simulink model "signal_generator"  (R2020b)
settings: Solver=VariableStepAuto  StartTime=0.0  StopTime=2048/(fs*8)  RelTol=1e-3
values from neighbouring files (symbols this model uses):
  aximm_bits = n_blocks * k    (= 800)    [setup.m]
  aximm_enable = 1    [setup.m]
  aximm_reset = 0    [setup.m]
  fs = 160e6    (= 160000000)    [setup.m]
  k = 80    [fixed_point_to_frame.m]    (also in setup.m)
libraries: hdlsllib x12, dspsigops x7, commblkcod2 x1, simulink x1, lib_rfsoc_fec x1
settings Model: SimulationMode=accelerator  Creator=ckb13136  LastModifiedBy=ckb13136
settings GRTTargetCC: RTWCAPISignals=on  RTWCAPIParams=on

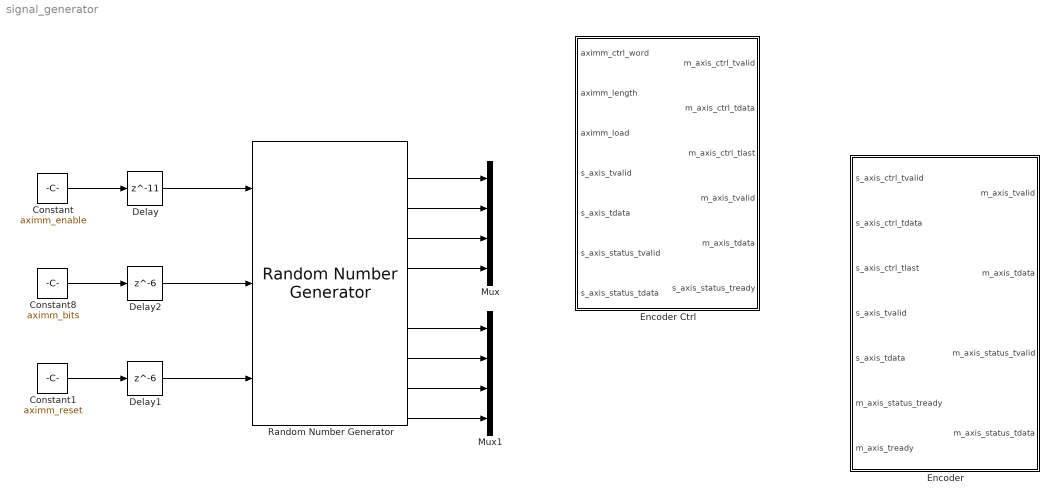
== system signal_generator ==
  Constant : Constant  Value=aximm_enable  OutDataTypeStr=uint32  SampleTime=1/fs
  Constant1 : Constant  Value=aximm_reset  OutDataTypeStr=uint32  SampleTime=1/fs
  Constant8 : Constant  Value=aximm_bits  OutDataTypeStr=uint32  SampleTime=1/fs
  Delay : Delay  DelayLength=11
  Delay1 : Delay  DelayLength=6
  Delay2 : Delay  DelayLength=6
  Encoder : Subsystem
  Encoder Ctrl : Subsystem  AncestorBlock=lib_rfsoc_fec/FEC Ctrl  TreatAsAtomicUnit=on
  Mux : Mux
  Mux1 : Mux
  Random Number Generator : lib_rfsoc_fec/Random Number Generator  SystemSampleTime=-1  VariantActivationTime=update diagram  Latency=0  AutoFrameSizeCalculation=off
  wires:
  Delay/1 -> Random Number Generator/1
  Constant8/1 -> Delay2/1
  Delay2/1 -> Random Number Generator/2
  Constant/1 -> Delay/1
  Delay1/1 -> Random Number Generator/3
  Constant1/1 -> Delay1/1
  Random Number Generator/2 -> Mux/1
  Random Number Generator/3 -> Mux/2
  Random Number Generator/4 -> Mux/3
  Random Number Generator/5 -> Mux/4
  Random Number Generator/7 -> Mux1/1
  Random Number Generator/8 -> Mux1/2
  Random Number Generator/9 -> Mux1/3
  Random Number Generator/10 -> Mux1/4

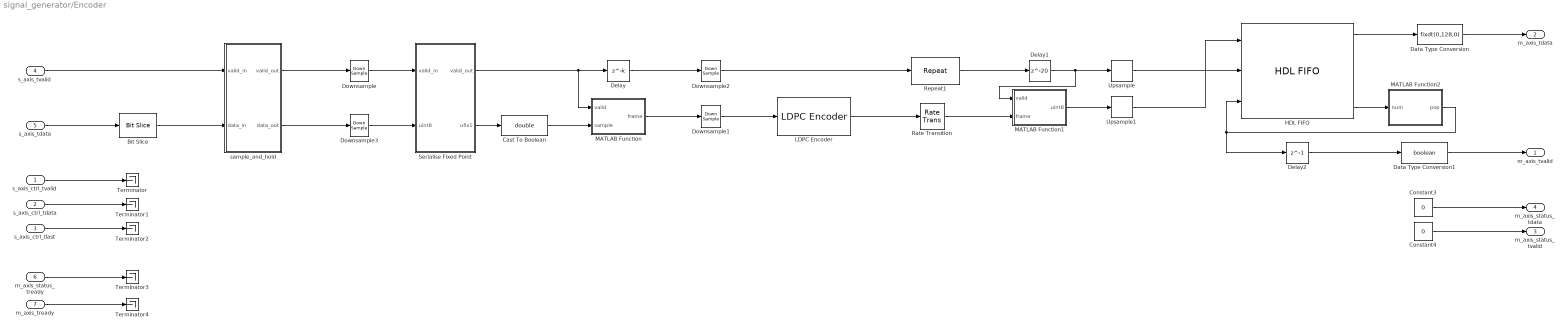
== system signal_generator/Encoder ==
  s_axis_ctrl_tvalid : Inport
  s_axis_ctrl_tdata : Inport  Port=2
  s_axis_ctrl_tlast : Inport  Port=3
  s_axis_tvalid : Inport  Port=4
  s_axis_tdata : Inport  Port=5
  m_axis_status_tready : Inport  Port=6
  m_axis_tready : Inport  Port=7
  Bit Slice : hdlsllib/Logic and Bit Operations/Bit Slice  lidx=7  ridx=0
      settings: SourceProductBaseCode=SL
  Cast To Boolean : DataTypeConversion  OutDataTypeStr=double
  Constant3 : Constant  Value=0  OutDataTypeStr=uint32  SampleTime=1/(fs*16)
  Constant4 : Constant  Value=0  OutDataTypeStr=boolean  SampleTime=1/(fs*16)
  Data Type Conversion : DataTypeConversion  OutDataTypeStr=fixdt(0,128,0)
  Data Type Conversion1 : DataTypeConversion  OutDataTypeStr=boolean
  Delay : Delay  DelayLength=k
  Delay1 : Delay  DelayLength=20
  Delay2 : Delay  DelayLength=1
  Downsample : DownSample  N=16  RateOptions=Allow multirate processing
  Downsample1 : DownSample  N=80  RateOptions=Allow multirate processing
  Downsample2 : DownSample  N=80  RateOptions=Allow multirate processing
  Downsample3 : DownSample  N=16  RateOptions=Allow multirate processing
  HDL FIFO : hdlsllib/HDL RAMs/HDL FIFO  fifo_size=8192  mode=Classic  ratio=1  push_msg=Warning  pop_msg=Warning  show_empty=on  show_full=on  show_num=on  LabelModeActiveChoice_Mode=Classic
      settings: SourceProductBaseCode=SL
  LDPC Encoder : commblkcod2/LDPC Encoder  ParityCheckMat=parity_sparse
      settings: SourceProductBaseCode=CM
  MATLAB Function : MATLAB Function  TreatAsAtomicUnit=on
  MATLAB Function1 : MATLAB Function  TreatAsAtomicUnit=on
  MATLAB Function2 : MATLAB Function  TreatAsAtomicUnit=on
  Rate Transition : RateTransition
  Repeat1 : dspsigops/Repeat  N=20  InputProcessing=Columns as channels (frame based)  RateOptions=Allow multirate processing  ic=0  mode=Unused parameter value
      settings: SourceProductName=DSP System Toolbox
  Serialise Fixed Point : Subsystem
  Terminator{,1..4} (5 alike) : Terminator
  Upsample : dspsigops/Upsample  N=8  phase=0  RateOptions=Allow multirate processing  ic=0  mode=Unused parameter value
  Upsample1 : dspsigops/Upsample  N=8  phase=0  RateOptions=Allow multirate processing  ic=0  mode=Unused parameter value
  sample_and_hold : Subsystem
  m_axis_tvalid : Outport
  m_axis_tdata : Outport  Port=2
  m_axis_status_tvalid : Outport  Port=3
  m_axis_status_tdata : Outport  Port=4
  wires:
  m_axis_tready/1 -> Terminator4/1
  Data Type Conversion1/1 -> m_axis_tvalid/1
  Delay2/1 -> Data Type Conversion1/1
  MATLAB Function2/1(pop) -> HDL FIFO/3, Delay2/1
  HDL FIFO/4 -> MATLAB Function2/1(num)
  Data Type Conversion/1 -> m_axis_tdata/1
  Upsample/1 -> HDL FIFO/2
  Upsample1/1 -> HDL FIFO/1
  HDL FIFO/1 -> Data Type Conversion/1
  Delay1/1 -> Upsample/1, MATLAB Function1/1(valid)
  Bit Slice/1 -> sample_and_hold/2(data_in)
  Rate Transition/1 -> MATLAB Function1/2(frame)
  LDPC Encoder/1 -> Rate Transition/1
  sample_and_hold/2(" data_out") -> Downsample3/1
  sample_and_hold/1(" valid_out") -> Downsample/1
  s_axis_tdata/1 -> Bit Slice/1
  s_axis_tvalid/1 -> sample_and_hold/1(valid_in)
  Downsample3/1 -> Serialise Fixed Point/2(uint8)
  m_axis_status_tready/1 -> Terminator3/1
  s_axis_ctrl_tlast/1 -> Terminator2/1
  s_axis_ctrl_tdata/1 -> Terminator1/1
  s_axis_ctrl_tvalid/1 -> Terminator/1
  Downsample/1 -> Serialise Fixed Point/1(valid_in)
  Downsample1/1 -> LDPC Encoder/1
  Delay/1 -> Downsample2/1
  Repeat1/1 -> Delay1/1
  MATLAB Function1/1(uint8) -> Upsample1/1
  MATLAB Function/1(frame) -> Downsample1/1
  Serialise Fixed Point/1(valid_out) -> MATLAB Function/1(valid), Delay/1
  Cast To Boolean/1 -> MATLAB Function/2(sample)
  Downsample2/1 -> Repeat1/1
  Constant4/1 -> m_axis_status_tvalid/1
  Constant3/1 -> m_axis_status_tdata/1
  Serialise Fixed Point/2(ufix1) -> Cast To Boolean/1

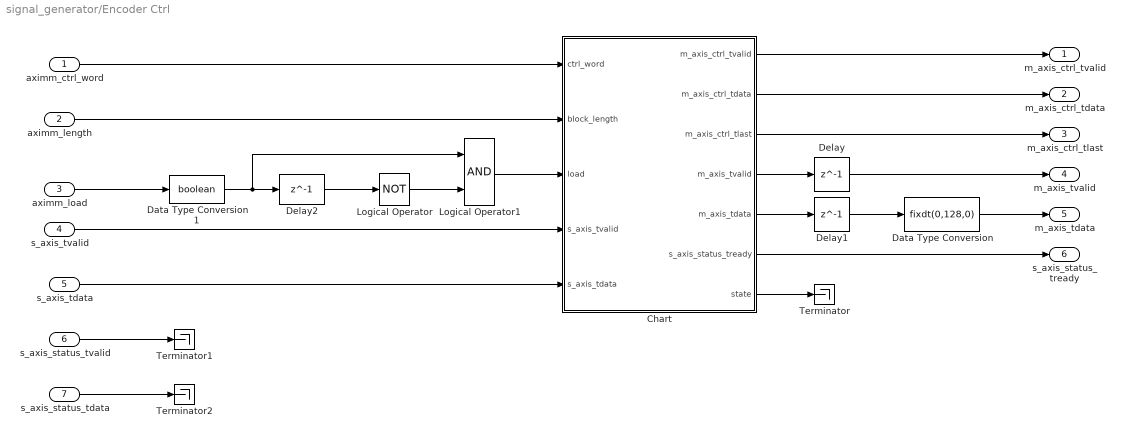
== system signal_generator/Encoder Ctrl ==
  aximm_ctrl_word : Inport
  aximm_length : Inport  Port=2
  aximm_load : Inport  Port=3
  s_axis_tvalid : Inport  Port=4
  s_axis_tdata : Inport  Port=5
  s_axis_status_tvalid : Inport  Port=6
  s_axis_status_tdata : Inport  Port=7
  Chart : Stateflow chart  TreatAsAtomicUnit=on
  Data Type Conversion : DataTypeConversion  OutDataTypeStr=fixdt(0,128,0)
  Data Type Conversion1 : DataTypeConversion  OutDataTypeStr=boolean  SaturateOnIntegerOverflow=on  RndMeth=Zero
  Delay : Delay  DelayLength=1
  Delay1 : Delay  DelayLength=1
  Delay2 : Delay  DelayLength=1  InitialCondition=1  InputProcessing=Columns as channels (frame based)
  Logical Operator : Logic  Operator=NOT  Inputs=1
  Logical Operator1 : Logic
  Terminator : Terminator
  Terminator1 : Terminator
  Terminator2 : Terminator
  m_axis_ctrl_tvalid : Outport
  m_axis_ctrl_tdata : Outport  Port=2
  m_axis_ctrl_tlast : Outport  Port=3
  m_axis_tvalid : Outport  Port=4
  m_axis_tdata : Outport  Port=5
  s_axis_status_tready : Outport  Port=6
  wires:
  Chart/3(m_axis_ctrl_tlast) -> m_axis_ctrl_tlast/1
  Chart/7(state) -> Terminator/1
  aximm_length/1 -> Chart/2(block_length)
  s_axis_tvalid/1 -> Chart/4(s_axis_tvalid)
  s_axis_tdata/1 -> Chart/5(s_axis_tdata)
  aximm_ctrl_word/1 -> Chart/1(ctrl_word)
  Chart/2(m_axis_ctrl_tdata) -> m_axis_ctrl_tdata/1
  Chart/4(m_axis_tvalid) -> Delay/1
  Chart/5(m_axis_tdata) -> Delay1/1
  Chart/6(s_axis_status_tready) -> s_axis_status_tready/1
  Chart/1(m_axis_ctrl_tvalid) -> m_axis_ctrl_tvalid/1
  Delay/1 -> m_axis_tvalid/1
  Delay1/1 -> Data Type Conversion/1
  Data Type Conversion/1 -> m_axis_tdata/1
  Logical Operator1/1 -> Chart/3(load)
  s_axis_status_tvalid/1 -> Terminator1/1
  s_axis_status_tdata/1 -> Terminator2/1
  Logical Operator/1 -> Logical Operator1/2
  Data Type Conversion1/1 -> Delay2/1, Logical Operator1/1
  Delay2/1 -> Logical Operator/1
  aximm_load/1 -> Data Type Conversion1/1

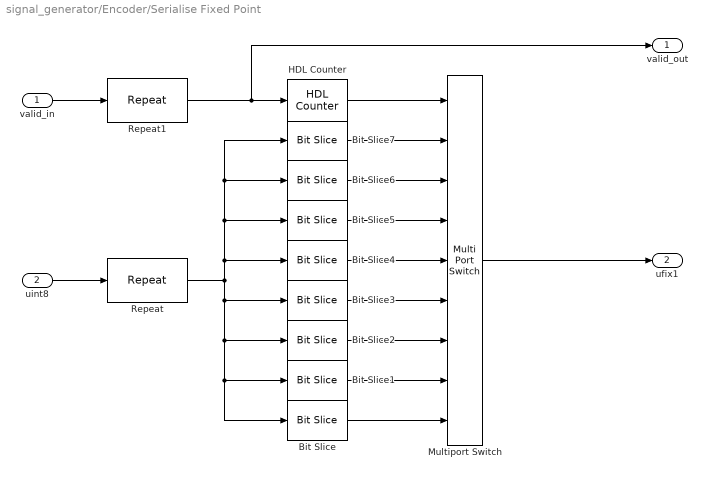
== system signal_generator/Encoder/Serialise Fixed Point ==
  valid_in : Inport
  uint8 : Inport  Port=2
  Bit Slice : hdlsllib/Logic and Bit Operations/Bit Slice  lidx=0  ridx=0
      settings: SourceProductBaseCode=SL
  Bit Slice1 : hdlsllib/Logic and Bit Operations/Bit Slice  lidx=1  ridx=1
      settings: SourceProductBaseCode=SL
  Bit Slice2 : hdlsllib/Logic and Bit Operations/Bit Slice  lidx=2  ridx=2
      settings: SourceProductBaseCode=SL
  Bit Slice3 : hdlsllib/Logic and Bit Operations/Bit Slice  lidx=3  ridx=3
      settings: SourceProductBaseCode=SL
  Bit Slice4 : hdlsllib/Logic and Bit Operations/Bit Slice  lidx=4  ridx=4
      settings: SourceProductBaseCode=SL
  Bit Slice5 : hdlsllib/Logic and Bit Operations/Bit Slice  lidx=5  ridx=5
      settings: SourceProductBaseCode=SL
  Bit Slice6 : hdlsllib/Logic and Bit Operations/Bit Slice  lidx=6  ridx=6
      settings: SourceProductBaseCode=SL
  Bit Slice7 : hdlsllib/Logic and Bit Operations/Bit Slice  lidx=7  ridx=7
      settings: SourceProductBaseCode=SL
  HDL Counter : hdlsllib/Sources/HDL Counter  CountType=Count limited  CountInit=7  CountStep=-1  CountMax=0  CountFromType=Initial value  CountFrom=7  CountResetPort=off  CountLoadPort=off  CountEnbPort=on  CountDirPort=off  CountDataType=Unsigned  CountWordLen=3  CountFracLen=0  CountSampTime=1
  Multiport Switch : MultiPortSwitch  DataPortOrder=Zero-based contiguous  Inputs=8  zeroidx=on
  Repeat : dspsigops/Repeat  N=8  InputProcessing=Columns as channels (frame based)  RateOptions=Allow multirate processing  ic=0  mode=Unused parameter value
      settings: SourceProductName=DSP System Toolbox
  Repeat1 : dspsigops/Repeat  N=8  InputProcessing=Columns as channels (frame based)  RateOptions=Allow multirate processing  ic=0  mode=Unused parameter value
      settings: SourceProductName=DSP System Toolbox
  valid_out : Outport
  ufix1 : Outport  Port=2
  wires:
  Multiport Switch/1 -> ufix1/1
  valid_in/1 -> Repeat1/1
  Bit Slice7/1 -> Multiport Switch/2
  HDL Counter/1 -> Multiport Switch/1
  Bit Slice3/1 -> Multiport Switch/6
  Bit Slice2/1 -> Multiport Switch/7
  Bit Slice1/1 -> Multiport Switch/8
  Bit Slice6/1 -> Multiport Switch/3
  Repeat1/1 -> HDL Counter/1, valid_out/1
  Bit Slice/1 -> Multiport Switch/9
  Bit Slice5/1 -> Multiport Switch/4
  Repeat/1 -> Bit Slice4/1, Bit Slice5/1, Bit Slice6/1, Bit Slice7/1, Bit Slice3/1, Bit Slice2/1, Bit Slice1/1, Bit Slice/1
  Bit Slice4/1 -> Multiport Switch/5
  uint8/1 -> Repeat/1

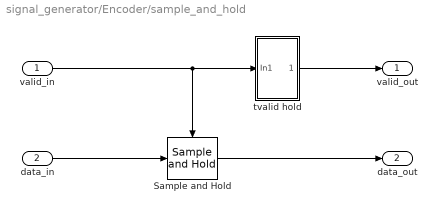
== system signal_generator/Encoder/sample_and_hold ==
  valid_in : Inport
  data_in : Inport  Port=2
  Sample and Hold : dspsigops/Sample and Hold  trig=Rising edge  initCond=0  latchinput=off
  tvalid hold : Subsystem
  " valid_out" : Outport
  " data_out" : Outport  Port=2
  wires:
  Sample and Hold/1 -> " data_out"/1
  data_in/1 -> Sample and Hold/1
  tvalid hold/1(" ") -> " valid_out"/1
  valid_in/1 -> Sample and Hold/Trigger, tvalid hold/1(In1)

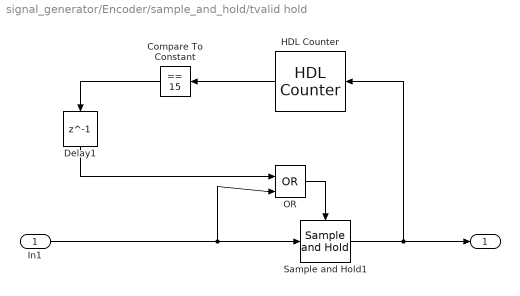
== system signal_generator/Encoder/sample_and_hold/tvalid hold ==
  In1 : Inport
  Compare To Constant : simulink/Logic and Bit Operations/Compare To Constant  relop===  const=15  OutDataTypeStr=boolean
  Delay1 : Delay  DelayLength=1
  HDL Counter : hdlsllib/Sources/HDL Counter  CountType=Count limited  CountInit=0  CountStep=1  CountMax=15  CountFromType=Initial value  CountFrom=0  CountResetPort=off  CountLoadPort=off  CountEnbPort=on  CountDirPort=off  CountDataType=Unsigned  CountWordLen=4  CountFracLen=0  CountSampTime=1
  OR : Logic  Operator=OR  IconShape=distinctive  AllPortsSameDT=off  OutDataTypeStr=boolean
  Sample and Hold1 : dspsigops/Sample and Hold  trig=Rising edge  initCond=0  latchinput=off
  " " : Outport
  wires:
  In1/1 -> OR/2, Sample and Hold1/1
  Sample and Hold1/1 -> HDL Counter/1, " "/1
  Compare To Constant/1 -> Delay1/1
  OR/1 -> Sample and Hold1/Trigger
  Delay1/1 -> OR/1
  HDL Counter/1 -> Compare To Constant/1

== matlab function signal_generator/Encoder/MATLAB Function ==
  data: valid input; sample input; frame output size=[80,1] [0..80]; k parameter
function frame = fcn(valid, sample, k)

persistent f count prev_frame

if isempty(f)
    f = zeros(1,80)';
    prev_frame = zeros(1,80)';
    count = 0;
end

frame = prev_frame;

if valid
    count = count + 1;
    f(count) = sample;
end

if count >= k
    prev_frame = f;
    count = 0;
end

== matlab function signal_generator/Encoder/MATLAB Function1 ==
  data: valid input; frame input; uint8 output [0..80]; k parameter
function uint8 = fcn(valid, frame, k)

persistent f u count

if isempty(f)
    f = zeros(1,8);
    u = fi(0,0,8,0);
    count = 0;
end

if valid
    f = frame((1:8)+(8*count));
    u(:) = f(8)*2^7 ...
      + f(7)*2^6 ...
      + f(6)*2^5 ...
      + f(5)*2^4 ...
      + f(4)*2^3 ...
      + f(3)*2^2 ...
      + f(2)*2^1 ...
      + f(1)*2^0;
  count = count + 1;
end

if count >= 20
    count = 0;
end

uint8 = u;

== matlab function signal_generator/Encoder/MATLAB Function2 ==
  data: num input; pop output [0..80]
function pop = fcn(num)

persistent count flag

if isempty(count)
    count = 0;
    flag = 0;
end

pop = 0;

if num == 20
    flag = 1;
end

if flag
    pop = 1;
    count = count + 1;
end

if count >= 20
    count = 0;
    flag = 0;
end

== stateflow chart signal_generator/Encoder Ctrl/Chart ==
  settings: executeAtInitialization=1
  state LOAD_NVALID
    % Local
    loaded_n(:) = block_length;
    loaded_ctrl(:) = ctrl_word;
    %
    % DATA Stream
    m_axis_tdata(:) = 0;
    m_axis_tvalid(:) = false;
    %
    % CTRL Stream
    m_axis_ctrl_tdata(:) = 0;
    m_axis_ctrl_tlast(:) = false;
    m_axis_ctrl_tvalid(:) = false;
    %
    % STATUS Stream
    s_axis_status_tready(:) = true;
  state LOAD_VALID
    % Local
    count(:) = count + 1;
    loaded_n(:) = block_length;
    loaded_ctrl(:) = ctrl_word;
    %
    % DATA Stream
    m_axis_tdata(:) = s_axis_tdata;
    m_axis_tvalid(:) = true;
    %
    % CTRL Stream
    m_axis_ctrl_tdata(:) = 0;
    m_axis_ctrl_tlast(:) = false;
    m_axis_ctrl_tvalid(:) = false;
    %
    % STATUS Stream
    s_axis_status_tready(:) = true;
  state IDLE
    % Local
    %
    % DATA Stream
    m_axis_tdata = fi(0,0,8,0);
    m_axis_tvalid = false;
    %
    % CTRL Stream
    m_axis_ctrl_tdata = fi(0,0,32,0);
    m_axis_ctrl_tlast = false;
    m_axis_ctrl_tvalid = false;
    %
    % STATUS Stream
    s_axis_status_tready = false;
  state INIT
    % Local
    count = fi(0,0,32,0);
    n = fi(0,0,32,0);
    loaded_n = fi(0,0,32,0);
    loaded_ctrl = fi(0,0,32,0);
    %
    % DATA Stream
    m_axis_tdata = fi(0,0,8,0);
    m_axis_tvalid = false;
    %
    % CTRL Stream
    m_axis_ctrl_tdata = fi(0,0,32,0);
    m_axis_ctrl_tlast = false;
    m_axis_ctrl_tvalid = false;
    %
    % STATUS Stream
    s_axis_status_tready = false;
  state CTRL
    % Local
    count(:) = count + 1;
    n(:) = loaded_n;
    %
    % DATA Stream
    m_axis_tdata(:) = s_axis_tdata;
    m_axis_tvalid(:) = true;
    %
    % CTRL Stream
    m_axis_ctrl_tdata(:) = loaded_ctrl;
    m_axis_ctrl_tlast(:) = true;
    m_axis_ctrl_tvalid(:) = true;
    %
    % STATUS Stream
    s_axis_status_tready(:) = true;
  state COUNT_DIN
    % Local
    count(:) = count + 1;
    %
    % DATA Stream
    m_axis_tdata(:) = s_axis_tdata;
    m_axis_tvalid(:) = true;        % Complete a full block
    %
    % CTRL Stream
    m_axis_ctrl_tdata(:) = 0;
    m_axis_ctrl_tlast(:) = false;
    m_axis_ctrl_tvalid(:) = false;
    %
    % STATUS Stream
    s_axis_status_tready(:) = true;
  state WAITING
    % Local
    %
    % DATA Stream
    m_axis_tdata(:) = s_axis_tdata;
    m_axis_tvalid(:) = false;
    %
    % CTRL Stream
    m_axis_ctrl_tdata(:) = 0;
    m_axis_ctrl_tlast(:) = false;
    m_axis_ctrl_tvalid(:) = false;
    %
    % STATUS Stream
    s_axis_status_tready(:) = true;
  LOAD_VALID -> IDLE [order 3] : [count >= n && s_axis_tvalid == 0]{count(:) = 0}
  (default) -> INIT
  LOAD_VALID -> CTRL [order 2] : [count >= n && s_axis_tvalid == 1]{count(:) = 0}
  LOAD_NVALID -> COUNT_DIN [order 2] : [s_axis_tvalid == 1 && count > 0]
  IDLE -> LOAD_NVALID [order 1] : [load == 1]
  INIT -> IDLE
  LOAD_VALID -> COUNT_DIN [order 1] : [count < n]
  CTRL -> LOAD_VALID [order 1] : [load == 1 && s_axis_tvalid == 1]
  COUNT_DIN -> LOAD_NVALID [order 5] : [load == 1 && s_axis_tvalid == 0]
  COUNT_DIN -> IDLE [order 3] : [count >= n && s_axis_tvalid == 0]{count(:) = 0}
  IDLE -> CTRL [order 2] : [s_axis_tvalid == 1 && count ==0]
  LOAD_NVALID -> CTRL [order 1] : [s_axis_tvalid == 1 && count ==0]
  COUNT_DIN -> LOAD_VALID [order 2] : [load == 1 && s_axis_tvalid == 1]
  COUNT_DIN -> WAITING [order 4] : [load == 0 && s_axis_tvalid == 0]
  CTRL -> COUNT_DIN [order 2] : [s_axis_tvalid == 1]
  COUNT_DIN -> CTRL [order 1] : [count >= n && s_axis_tvalid == 1]{count(:) = 0}
  WAITING -> COUNT_DIN : [s_axis_tvalid == 1]
  CTRL -> WAITING [order 3] : [s_axis_tvalid == 0]
  data: m_axis_ctrl_tvalid output; ctrl_word input; count local; m_axis_ctrl_tdata output; m_axis_ctrl_tlast output; m_axis_tvalid output; block_length input; load input; s_axis_tvalid input; m_axis_tdata output; s_axis_tdata input; s_axis_status_tready output; n local; loaded_ctrl local; loaded_n local; state output Enum: stateType
